simulink model "NOLCO1"  (R2017a)
settings: Solver=VariableStepAuto  StartTime=0.0  StopTime=20.0  RelTol=1e-3
values from neighbouring files (symbols this model uses):
  epsilon = 1e-3    (= 0.001)    [config1.m]
  omega = 5    [config1.m]
  omega_z = 5    [config1.m]
  psi = 1    [config1.m]
  psi_z = 1    [config1.m]
settings Model: Creator=lbergantin2017  LastModifiedBy=lbergantin2017

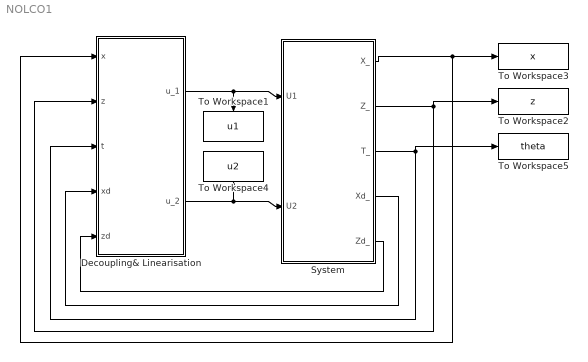
== system NOLCO1 ==
  Decoupling& Linearisation : Subsystem
  System : Subsystem
  To Workspace1 : ToWorkspace  VariableName=u1  SampleTime=-1
  To Workspace2 : ToWorkspace  VariableName=z  SampleTime=-1
  To Workspace3 : ToWorkspace  VariableName=x  SampleTime=-1
  To Workspace4 : ToWorkspace  VariableName=u2  SampleTime=-1
  To Workspace5 : ToWorkspace  VariableName=theta  SampleTime=-1
  wires:
  Decoupling& Linearisation/1(u_1) -> System/1("U1 "), To Workspace1/1
  System/1(X_) -> To Workspace3/1, Decoupling& Linearisation/1(x)
  System/2("Z_ ") -> To Workspace2/1, Decoupling& Linearisation/2(z)
  Decoupling& Linearisation/2(u_2) -> To Workspace4/1, System/2(U2)
  System/3(T_) -> To Workspace5/1, Decoupling& Linearisation/3("t ")
  System/4(Xd_) -> Decoupling& Linearisation/4(xd)
  System/5(Zd_) -> Decoupling& Linearisation/5(zd)

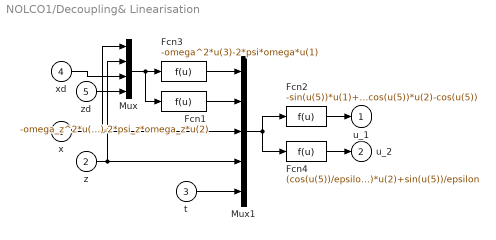
== system NOLCO1/Decoupling& Linearisation ==
  x : Inport
  z : Inport  Port=2
  "t " : Inport  Port=3
  xd : Inport  Port=4
  zd : Inport  Port=5
  Fcn1 : Fcn  Expr=-omega_z^2*u(4)-2*psi_z*omega_z*u(2)
  Fcn2 : Fcn  Expr=-sin(u(5))*u(1)+cos(u(5))*u(2)-cos(u(5))
  Fcn3 : Fcn  Expr=-omega^2*u(3)-2*psi*omega*u(1)
  Fcn4 : Fcn  Expr=(cos(u(5))/epsilon)*u(1)+(sin(u(5))/epsilon)*u(2)+sin(u(5))/epsilon
  Mux : Mux
  Mux1 : Mux  Inputs=5
  u_1 : Outport
  u_2 : Outport  Port=2
  wires:
  x/1 -> Mux/1, Mux1/3
  Fcn3/1 -> Mux1/1
  Fcn2/1 -> u_1/1
  "t "/1 -> Mux1/5
  xd/1 -> Mux/3
  zd/1 -> Mux/4
  Mux/1 -> Fcn1/1, Fcn3/1
  Mux1/1 -> Fcn2/1, Fcn4/1
  Fcn4/1 -> u_2/1
  Fcn1/1 -> Mux1/2
  z/1 -> Mux1/4, Mux/2

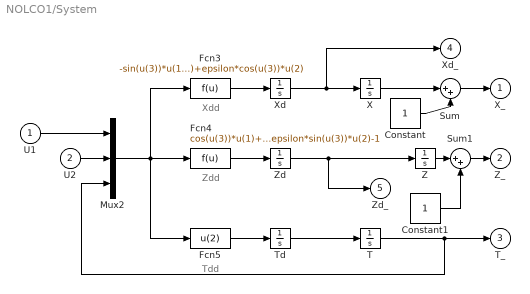
== system NOLCO1/System ==
  note: Xdd
  note: Zdd
  note: Tdd
  "U1 " : Inport
  U2 : Inport  Port=2
  Constant : Constant
  Constant1 : Constant
  Fcn3 : Fcn  Expr=-sin(u(3))*u(1)+epsilon*cos(u(3))*u(2)
  Fcn4 : Fcn  Expr=cos(u(3))*u(1)+epsilon*sin(u(3))*u(2)-1
  Fcn5 : Fcn  Expr=u(2)
  Mux2 : Mux  Inputs=3
  Sum : Sum  Inputs=|++
  Sum1 : Sum  Inputs=|++
  T : Integrator
  Td : Integrator
  X : Integrator
  Xd : Integrator
  Z : Integrator
  Zd : Integrator
  X_ : Outport
  "Z_ " : Outport  Port=2
  T_ : Outport  Port=3
  Xd_ : Outport  Port=4
  Zd_ : Outport  Port=5
  wires:
  Fcn3/1 -> Xd/1
  Xd/1 -> Xd_/1, X/1
  Zd/1 -> Zd_/1, Z/1
  Fcn4/1 -> Zd/1
  Fcn5/1 -> Td/1
  Mux2/1 -> Fcn5/1, Fcn3/1, Fcn4/1
  Td/1 -> T/1
  X/1 -> Sum/1
  "U1 "/1 -> Mux2/1
  U2/1 -> Mux2/2
  T/1 -> Mux2/3, T_/1
  Sum/1 -> X_/1
  Constant/1 -> Sum/2
  Z/1 -> Sum1/1
  Sum1/1 -> "Z_ "/1
  Constant1/1 -> Sum1/2
